simulink model "uncontrolled_case"  (R2020b)
settings: Solver=ode15s  StartTime=0.0  StopTime=T  MaxStep=0.01  RelTol=1e-3
values from neighbouring files (symbols this model uses):
  a1A = 0.5    [sim_D_FB_J.m]
  a1B = 0.5    [sim_D_FB_J.m]
  a2A = 0.5    [sim_D_FB_J.m]
  a2B = 0.5    [sim_D_FB_J.m]
  a3A = 0.5    [sim_D_FB_J.m]
  a3B = 0.5    [sim_D_FB_J.m]
  friction = [fv1p fv2p fv1A fv2A fv3A fv1B fv2B fv3B]    [sim_second_arm_compensation.m]    (also in sim_second_arm_compensation2.m; sim_second_arm_compensation3.m)
  fv1A = 0    [sim_D_FB_J.m]
  fv1B = 0    [sim_D_FB_J.m]
  fv2A = 0    [sim_D_FB_J.m]
  fv2B = 0    [sim_D_FB_J.m]
  fv3A = 0    [sim_D_FB_J.m]
  fv3B = 0    [sim_D_FB_J.m]
  g = [0 -g0 0]'    [sim_second_arm_compensation.m]    (also in sim_second_arm_compensation2.m; sim_second_arm_compensation3.m)
  info = struct('n_joints', n_joints,                'n_links', n_links,                'n_ee', n_ee,                'current_frame_index',    [1  2 3 4 5 6 7  8 9 10],                'previous_frame_index',   [0  1 2 3 4 2 6  7 5  8],                'next_frame_index',       [2 36 4 5 9 7 8 10 0  0],                'next_frame_type',        [0  1 0 0 0 0 0  0 0  0],                'previous_joint_index',  ...(+449 chars)    [sim_second_arm_compensation.m]    (also in sim_second_arm_compensation2.m; sim_second_arm_compensation3.m)
  Kd = 5*eye(6)    [sim_D_FB_J.m]    (also in sim_second_arm_compensation.m; sim_second_arm_compensation2.m; sim_second_arm_compensation3.m = diag([5 5 5 1 1 1]))
  Kp = 5*eye(6)    [sim_D_FB_J.m]    (also in sim_second_arm_compensation.m; sim_second_arm_compensation2.m; sim_second_arm_compensation3.m = diag([5 5 5 1 1 1]))
  L = 3    [sim_D_FB_J.m]
  m_base = 100    [sim_D_FB_J.m]
  m_cavo = 45    [sim_D_FB_J.m]
  ml1A = 5    [sim_D_FB_J.m]
  ml1B = 5    [sim_D_FB_J.m]
  ml2A = 5    [sim_D_FB_J.m]
  ml2B = 5    [sim_D_FB_J.m]
  ml3A = 5    [sim_D_FB_J.m]
  ml3B = 5    [sim_D_FB_J.m]
  offA = -0.25    [sim_D_FB_J.m]
  offB = 0.25    [sim_D_FB_J.m]
  th1A_0 = -pi/2    (= -1.57079632679)    [sim_D_FB_J.m]    (also in sim_second_arm_compensation.m = 0; sim_second_arm_compensation2.m = 0; sim_second_arm_compensation3.m = -0.523598775598)
  th1B_0 = -pi/2    (= -1.57079632679)    [sim_D_FB_J.m]    (also in sim_second_arm_compensation.m = 0; sim_second_arm_compensation2.m = 0; sim_second_arm_compensation3.m = 0.523598775598)
  th2A_0 = -pi/8    (= -0.392699081699)    [sim_D_FB_J.m]    (also in sim_second_arm_compensation.m; sim_second_arm_compensation2.m; sim_second_arm_compensation3.m = 0.523598775598)
  th2B_0 = pi/8    (= 0.392699081699)    [sim_D_FB_J.m]    (also in sim_second_arm_compensation.m; sim_second_arm_compensation2.m; sim_second_arm_compensation3.m = -0.523598775598)
  th3A_0 = -pi/8    (= -0.392699081699)    [sim_D_FB_J.m]    (also in sim_second_arm_compensation.m; sim_second_arm_compensation2.m; sim_second_arm_compensation3.m = 0.523598775598)
  th3B_0 = pi/8    (= 0.392699081699)    [sim_D_FB_J.m]    (also in sim_second_arm_compensation.m; sim_second_arm_compensation2.m; sim_second_arm_compensation3.m = -0.523598775598)
undefined symbols (not defined in the file or in its folder): D, m_cables, m_carroponte, m_crane, m_platform, X, Y, Z
libraries: sm_lib x173, nesl_utility x62
(part 1 of 4)
settings Model: Creator=giank  LastModifiedBy=giank
settings ExplorerConfigSet: InternalSimMechanicsExplorerSettings="<ExplorerConfiguration><canonicalview>default</canonicalview><AnimationSetting><BasePlaybackSpeed>1.0</BasePlaybackSpeed><PlaybackSpeedFactor>1.0</PlaybackSpeedFactor></AnimationSetting><TilePanel><TileInfo><Tiles Columns=\"1\" Count=\"1\" Rows=\"1\"><Column Weight=\"1\"/><Row Weight=\"1\"/><Tile Height=\"1\" Width=\"1\" X=\"0\" Y=\"0\"/></Tiles></TileInfo><SceneInfo><SceneViewer><BGColor><R>0.60000002384185791</R><G>0.60000002384185791</G><B>0.60000002384185791</B></BGColor><Camera><DoPerspective>off</DoPerspective><Position><X>0</X><Y>-2.20697786868344448</Y><Z>3.0855161704941283</Z></Position><Center><X>0</X><Y>-2.20697786868344448</Y><Z>9.61255199882771194e-08</Z></Center><Up><X>0</X><Y>1</Y><Z>-0</Z></Up><ViewLimDist>1</ViewLimDist><YLim>2.29378715991973881</YLim><XLim>3.51908945507964566</XLim></Camera></SceneViewer></SceneInfo></TilePanel><MechEditorPanel><Cameras/><GfxPanelCameraMap/><VideoCreator><PlaybackSpeedRatio>1.0</PlaybackSpeedRatio><FrameRate>30</FrameRate><VideoFormat>Motion JPEG AVI</VideoFormat><FrameSize>auto</FrameSize></VideoCreator></MechEditorPanel></ExplorerConfiguration>"

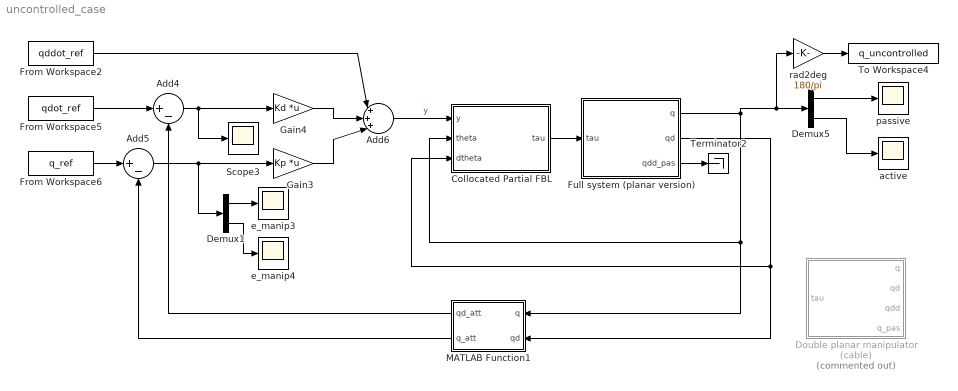
== system uncontrolled_case ==
  Add4 : Sum  Inputs=|+-
  Add5 : Sum  Inputs=|+-
  Add6 : Sum  Inputs=|+++|
  Collocated Partial FBL : MATLAB Function  TreatAsAtomicUnit=on
  Demux1 : Demux  Outputs=[3 3]
  Demux5 : Demux  Outputs=[2 6]
  Double planar manipulator (cable) : Subsystem  Commented=on
  From Workspace2 : FromWorkspace  VariableName=qddot_ref
  From Workspace5 : FromWorkspace  VariableName=qdot_ref
  From Workspace6 : FromWorkspace  VariableName=q_ref
  Full system (planar version) : Subsystem
  Gain3 : Gain  Gain=Kp  Multiplication=Matrix(K*u)
  Gain4 : Gain  Gain=Kd  Multiplication=Matrix(K*u)
  MATLAB Function1 : MATLAB Function  TreatAsAtomicUnit=on
  Scope3 : Scope
  Terminator2 : Terminator
  To Workspace4 : ToWorkspace  VariableName=q_uncontrolled  SaveFormat=Timeseries  SampleTime=-1
  active : Scope
  e_manip3 : Scope
  e_manip4 : Scope
  passive : Scope
  rad2deg : Gain  Gain=180/pi
  wires:
  From Workspace5/1 -> Add4/1
  MATLAB Function1/1(qd_att) -> Add4/2
  From Workspace6/1 -> Add5/1
  Add4/1 -> Scope3/1, Gain4/1
  Gain3/1 -> Add6/3
  Gain4/1 -> Add6/2
  Collocated Partial FBL/1(tau) -> Full system (planar version)/1(tau)
  MATLAB Function1/2(q_att) -> Add5/2
  Full system (planar version)/2(qd) -> Collocated Partial FBL/3(dtheta), MATLAB Function1/2(qd)
  Demux5/2 -> active/1
  Full system (planar version)/3(qdd_pas) -> Terminator2/1
  From Workspace2/1 -> Add6/1
  Demux5/1 -> passive/1
  Add6/1 -> Collocated Partial FBL/1(y)  "y"
  Full system (planar version)/1(q) -> rad2deg/1, Demux5/1, MATLAB Function1/1(q), Collocated Partial FBL/2(theta)
  Demux1/1 -> e_manip3/1
  Demux1/2 -> e_manip4/1
  Add5/1 -> Demux1/1, Gain3/1
  rad2deg/1 -> To Workspace4/1

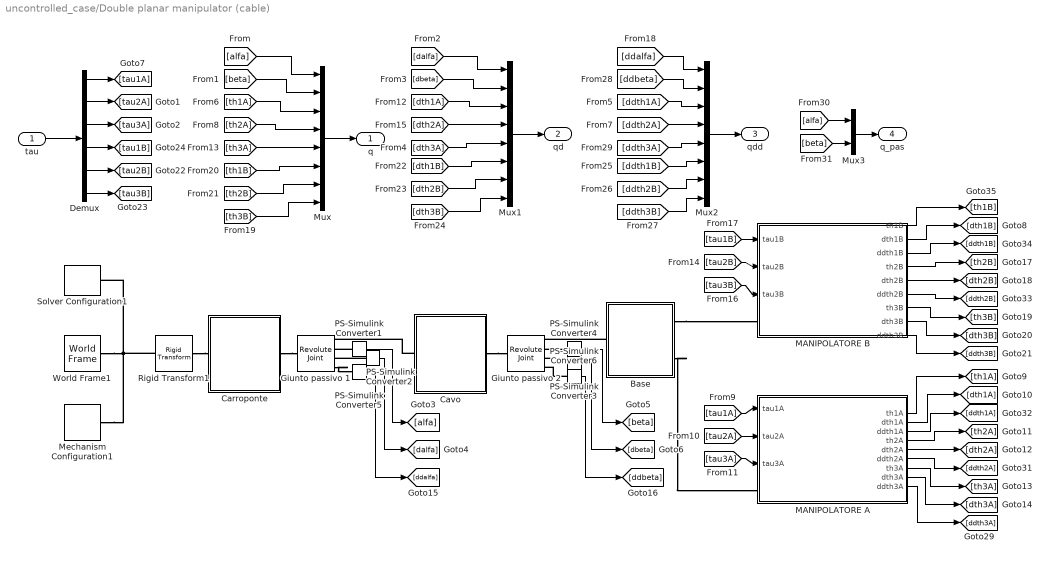
== system uncontrolled_case/Double planar manipulator (cable) ==
  tau : Inport
  Base : Subsystem  mask{L=1.2, W=0.15, H=0.15, m=m_base, rgb=[0.80 0.45 0]}
      mask prompts: L "Lenght (m)"; W "Width (m)"; H "Thickness (m)"; m "Mass (kg)"; rgb "Color [R G B]"
  Carroponte : Subsystem
  Cavo : Subsystem  mask{L=L, W=0.05, H=0.05, m=m_cavo, rgb=[0.3 0.3 0.3]}
      mask prompts: L "Lenght (m)"; W "Width (m)"; H "Thickness (m)"; m "Mass (kg)"; rgb "Color [R G B]"
  Demux : Demux  Outputs=6
  Giunto passivo 1 : sm_lib/Joints/Revolute Joint  JointMode=Normal  SenseConstraintForce=off  SenseConstraintForceX=off  SenseConstraintForceY=off  SenseConstraintForceZ=off  SenseConstraintTorque=off  SenseConstraintTorqueX=off  SenseConstraintTorqueY=off  SenseConstraintTorqueZ=off  SenseTotalForce=off  SenseTotalForceX=off  SenseTotalForceY=off  SenseTotalForceZ=off  SenseTotalTorque=off  SenseTotalTorqueX=off  SenseTotalTorqueY=off  SenseTotalTorqueZ=off  CompositeWrenchDir=FollowerOnBase  CompositeWrenchFrame=BaseFrame  EquilibriumPosition=0  EquilibriumPositionUnits=deg  SpringStiffness=0  SpringStiffnessUnits=N*m/deg  DampingCoefficient=fv1p  DampingCoefficientUnits=N*m/(rad/s)  TorqueActuationMode=NoTorque  MotionActuationMode=ComputedMotion  SensePosition=on  SenseVelocity=on  SenseAcceleration=on  SenseTorqueForce=off  SenseLowerLimitTorqueForce=off  SenseUpperLimitTorqueForce=off  LowerLimitSpecify=off  LowerLimitBound=-90  LowerLimitBoundUnits=deg  LowerLimitStiffness=1e4  LowerLimitStiffnessUnits=N*m/deg  LowerLimitDamping=10  LowerLimitDampingUnits=N*m/(deg/s)  LowerLimitTransitionRegionWidth=0.1  LowerLimitTransitionRegionWidthUnits=deg  UpperLimitSpecify=off  UpperLimitBound=90  UpperLimitBoundUnits=deg  UpperLimitStiffness=1e4  UpperLimitStiffnessUnits=N*m/deg  UpperLimitDamping=10  UpperLimitDampingUnits=N*m/(deg/s)  UpperLimitTransitionRegionWidth=0.1  UpperLimitTransitionRegionWidthUnits=deg  PositionTargetSpecify=on  PositionTargetPriority=High  PositionTargetValue=alfa_0  PositionTargetValueUnits=rad  VelocityTargetSpecify=off  VelocityTargetPriority=High  VelocityTargetValue=0  VelocityTargetValueUnits=deg/s
  Giunto passivo 2 : sm_lib/Joints/Revolute Joint  JointMode=Normal  SenseConstraintForce=off  SenseConstraintForceX=off  SenseConstraintForceY=off  SenseConstraintForceZ=off  SenseConstraintTorque=off  SenseConstraintTorqueX=off  SenseConstraintTorqueY=off  SenseConstraintTorqueZ=off  SenseTotalForce=off  SenseTotalForceX=off  SenseTotalForceY=off  SenseTotalForceZ=off  SenseTotalTorque=off  SenseTotalTorqueX=off  SenseTotalTorqueY=off  SenseTotalTorqueZ=off  CompositeWrenchDir=FollowerOnBase  CompositeWrenchFrame=BaseFrame  EquilibriumPosition=0  EquilibriumPositionUnits=deg  SpringStiffness=0  SpringStiffnessUnits=N*m/deg  DampingCoefficient=fv2p  DampingCoefficientUnits=N*m/(rad/s)  TorqueActuationMode=NoTorque  MotionActuationMode=ComputedMotion  SensePosition=on  SenseVelocity=on  SenseAcceleration=on  SenseTorqueForce=off  SenseLowerLimitTorqueForce=off  SenseUpperLimitTorqueForce=off  LowerLimitSpecify=off  LowerLimitBound=-90  LowerLimitBoundUnits=deg  LowerLimitStiffness=1e4  LowerLimitStiffnessUnits=N*m/deg  LowerLimitDamping=10  LowerLimitDampingUnits=N*m/(deg/s)  LowerLimitTransitionRegionWidth=0.1  LowerLimitTransitionRegionWidthUnits=deg  UpperLimitSpecify=off  UpperLimitBound=90  UpperLimitBoundUnits=deg  UpperLimitStiffness=1e4  UpperLimitStiffnessUnits=N*m/deg  UpperLimitDamping=10  UpperLimitDampingUnits=N*m/(deg/s)  UpperLimitTransitionRegionWidth=0.1  UpperLimitTransitionRegionWidthUnits=deg  PositionTargetSpecify=on  PositionTargetPriority=High  PositionTargetValue=beta_0  PositionTargetValueUnits=rad  VelocityTargetSpecify=off  VelocityTargetPriority=High  VelocityTargetValue=0  VelocityTargetValueUnits=deg/s
  MANIPOLATORE A : Subsystem  mask{th1_0=th1A_0, th2_0=th2A_0, th3_0=th3A_0, fv1=fv1A, fv2=fv2A, fv3=fv3A, a1=a1A, a2=a2A, a3=a3A, ml1=ml1A, ml2=ml2A, ml3=ml3A}
      mask prompts: th1_0 "th1_0 (rad)"; th2_0 "th2_0 (rad)"; th3_0 "th3_0 (rad)"; fv1 "Damping coeff. joint 1 (N*m/(rad/s))"; fv2 "Damping coeff. joint 2 (N*m/(rad/s))"; fv3 "Damping coeff. joint 3 (N*m/(rad/s))"; a1 "a1 (m)"; a2 "a2 (m)"; a3 "a3 (m)"; ml1 "ml1 (kg)"; ml2 "ml2 (kg)"; ml3 "ml3 (kg)"
  MANIPOLATORE B : Subsystem  mask{th1_0=th1B_0, th2_0=th2B_0, th3_0=th3B_0, fv1=fv1B, fv2=fv2B, fv3=fv3B, a1=a1B, a2=a2B, a3=a3B, ml1=ml1B, ml2=ml2B, ml3=ml3B}
      mask prompts: th1_0 "th1_0 (rad)"; th2_0 "th2_0 (rad)"; th3_0 "th3_0 (rad)"; fv1 "Damping coeff. joint 1 (N*m/(rad/s))"; fv2 "Damping coeff. joint 2 (N*m/(rad/s))"; fv3 "Damping coeff. joint 3 (N*m/(rad/s))"; a1 "a1 (m)"; a2 "a2 (m)"; a3 "a3 (m)"; ml1 "ml1 (kg)"; ml2 "ml2 (kg)"; ml3 "ml3 (kg)"
  Mechanism Configuration1 : sm_lib/Utilities/Mechanism Configuration  UniformGravity=Constant  GravityVector=[0 -9.81 0]  GravityVectorUnits=m/s^2  GravityUnits=m/s^2  LinearizationDelta=0.001  JointModeTransitionNonlinearIterations=2
  Mux : Mux  Inputs=8
  Mux1 : Mux  Inputs=8
  Mux2 : Mux  Inputs=8
  Mux3 : Mux  Inputs=2
  PS-Simulink Converter{1..6} (6 alike) : nesl_utility/PS-Simulink Converter  PhysicalDomain=network_engine_domain  SubClassName=ps_output  LeftPortType=input  RightPortType=output  PseudoPeriodic=off  Frequencies=[]  Unit=inherit  AffineConversion=off
  Rigid Transform1 : sm_lib/Frames and Transforms/Rigid Transform  TranslationMethod=StandardAxis  TranslationStandardOffset=9.5  TranslationLengthUnit=cm  TranslationStandardAxis=-Y  TranslationCartesianOffset=[0 0 0]  TranslationROffset=0  TranslationROffsetUnits=m  TranslationZOffset=0  TranslationZOffsetUnits=m  TranslationThetaOffset=0  TranslationThetaOffsetUnits=deg  RotationMethod=StandardAxis  RotationAngleUnits=deg  RotationStandardAxis=+Y  RotationAngle=90  RotationArbitraryAxis=[0 0 1]  FollAlignAxisA=+X  BaseAlignAxisA=+Y  FollAlignAxisB=+Y  BaseAlignAxisB=+Z  RotationSequenceAxes=FollowerAxes  RotationSequence=XYX  RotationSequenceAngles=[0 0 0]  RotationSequenceAnglesUnits=deg  RotationMatrix=[1 0 0; 0 1 0; 0 0 1]
  Solver Configuration1 : nesl_utility/Solver Configuration  PhysicalDomain=network_engine_domain  SubClassName=solver  LeftPortType=input  RightPortType=generic  Tones=[]  Harmonics=[]  SimulateNoise=off  Profile=off  UseLocalSampling=off  EnableSwitchedLinearOptims=on  FrequencyDomain=off  UseCCode=off  RelTol=0.001  AbsTol=1e-06  MinStep=1e-09  ToWorkspace=off  RevertToSquareIcSolve=off  NumHomotopyIterations=100  PhasorMode=off  PhasorModeNumHarmonics=1  DoDC=off  ResidualTolerance=1e-09  UseLocalSolver=off  LocalSolverChoice=NE_BACKWARD_EULER_ADVANCER  LocalSolverSampleTime=0.001  DoFixedCost=off  MaxNonlinIter=3  MaxModeIter=2  ComputeImpulses=off  ImpulseIterations=2  LinearAlgebra=Sparse  EquationFormulation=NE_TIME_EF  DelaysMemoryBudget=1024  AutomaticFiltering=on  FilteringTimeConstant=0.001  PartitionStorageMethod=AS_NEEDED  PartitionMemoryBudget=1024  PartitionMethod=FAST
  World Frame1 : sm_lib/Frames and Transforms/World Frame
  q : Outport
  qd : Outport  Port=2
  qdd : Outport  Port=3
  q_pas : Outport  Port=4
  wires:
  Mux/1 -> q/1
  PS-Simulink Converter1/1 -> [alfa]
  PS-Simulink Converter2/1 -> [dalfa]
  PS-Simulink Converter4/1 -> [beta]
  PS-Simulink Converter3/1 -> [dbeta]
  tau/1 -> Demux/1
  Mux1/1 -> qd/1
  Demux/1 -> [tau1A]
  Demux/3 -> [tau3A]
  Demux/2 -> [tau2A]
  Demux/4 -> [tau1B]
  Demux/5 -> [tau2B]
  [beta] -> Mux/2
  [alfa] -> Mux/1
  [th1A] -> Mux/3
  [th2A] -> Mux/4
  [th3A] -> Mux/5
  [th1B] -> Mux/6
  [th2B] -> Mux/7
  [th3B] -> Mux/8
  [dalfa] -> Mux1/1
  [dbeta] -> Mux1/2
  [dth1A] -> Mux1/3
  [dth2A] -> Mux1/4
  [dth3A] -> Mux1/5
  [dth1B] -> Mux1/6
  [dth2B] -> Mux1/7
  [dth3B] -> Mux1/8
  Demux/6 -> [tau3B]
  PS-Simulink Converter5/1 -> [ddalfa]
  PS-Simulink Converter6/1 -> [ddbeta]
  [ddalfa] -> Mux2/1
  Mux2/1 -> qdd/1
  [ddth1A] -> Mux2/3
  [ddth3B] -> Mux2/8
  [ddth2B] -> Mux2/7
  [ddth2A] -> Mux2/4
  [ddbeta] -> Mux2/2
  [ddth1B] -> Mux2/6
  [ddth3A] -> Mux2/5
  [alfa] -> Mux3/1
  [beta] -> Mux3/2
  Mux3/1 -> q_pas/1
  MANIPOLATORE A/1(th1A) -> [th1A]
  [tau3B] -> MANIPOLATORE B/3(tau3B)
  MANIPOLATORE B/1(th1B) -> [th1B]
  [tau1B] -> MANIPOLATORE B/1(tau1B)
  [tau2B] -> MANIPOLATORE B/2(tau2B)
  MANIPOLATORE B/4(th2B) -> [th2B]
  MANIPOLATORE B/5(dth2B) -> [dth2B]
  MANIPOLATORE B/7(th3B) -> [th3B]
  MANIPOLATORE A/5(dth2A) -> [dth2A]
  [tau2A] -> MANIPOLATORE A/2(tau2A)
  MANIPOLATORE A/4(th2A) -> [th2A]
  MANIPOLATORE A/8(dth3A) -> [dth3A]
  MANIPOLATORE A/9(ddth3A) -> [ddth3A]
  MANIPOLATORE B/6(ddth2B) -> [ddth2B]
  [tau1A] -> MANIPOLATORE A/1(tau1A)
  MANIPOLATORE A/7(th3A) -> [th3A]
  MANIPOLATORE B/8(dth3B) -> [dth3B]
  MANIPOLATORE B/9(ddth3B) -> [ddth3B]
  MANIPOLATORE A/2(dth1A) -> [dth1A]
  MANIPOLATORE A/6(ddth2A) -> [ddth2A]
  [tau3A] -> MANIPOLATORE A/3(tau3A)
  MANIPOLATORE B/2(dth1B) -> [dth1B]
  MANIPOLATORE B/3(ddth1B) -> [ddth1B]
  MANIPOLATORE A/3(ddth1A) -> [ddth1A]
  connections:
  Rigid Transform1/LConn1 -- Mechanism Configuration1/RConn1 -- World Frame1/RConn1 -- Solver Configuration1/RConn1
  Cavo/LConn1 -- Giunto passivo 1/RConn1
  Rigid Transform1/RConn1 -- Carroponte/LConn1
  Carroponte/RConn1 -- Giunto passivo 1/LConn1
  Cavo/RConn1 -- Giunto passivo 2/LConn1
  Base/LConn1 -- Giunto passivo 2/RConn1
  PS-Simulink Converter1/LConn1 -- Giunto passivo 1/RConn2
  PS-Simulink Converter4/LConn1 -- Giunto passivo 2/RConn2
  PS-Simulink Converter3/LConn1 -- Giunto passivo 2/RConn3
  PS-Simulink Converter2/LConn1 -- Giunto passivo 1/RConn3
  Giunto passivo 1/RConn4 -- PS-Simulink Converter5/LConn1
  PS-Simulink Converter6/LConn1 -- Giunto passivo 2/RConn4
  Base/RConn1 -- MANIPOLATORE B/LConn1
  Base/RConn2 -- MANIPOLATORE A/LConn1

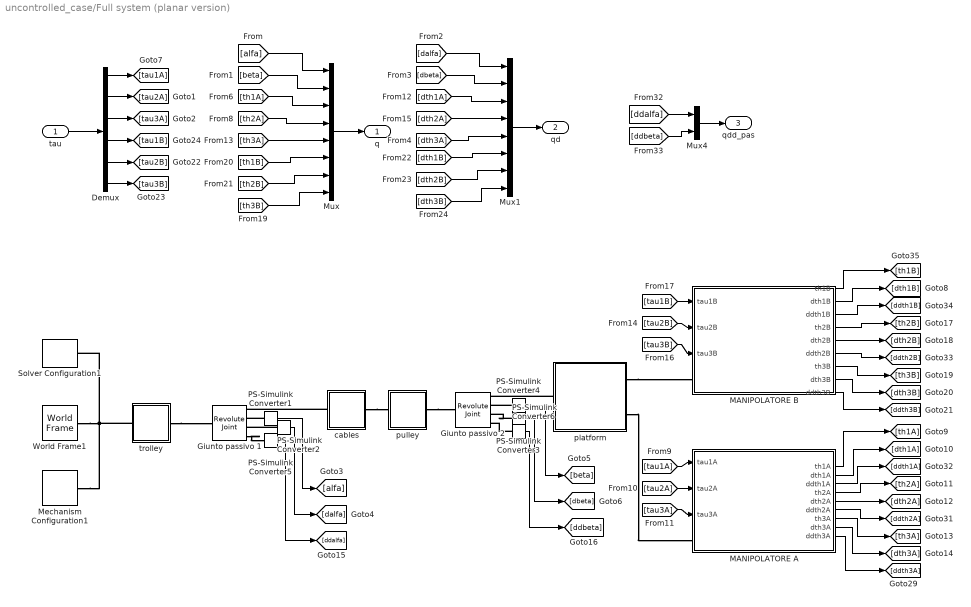
== system uncontrolled_case/Full system (planar version) ==
  tau : Inport
  Demux : Demux  Outputs=6
  Giunto passivo 1 : sm_lib/Joints/Revolute Joint  JointMode=Normal  SenseConstraintForce=off  SenseConstraintForceX=off  SenseConstraintForceY=off  SenseConstraintForceZ=off  SenseConstraintTorque=off  SenseConstraintTorqueX=off  SenseConstraintTorqueY=off  SenseConstraintTorqueZ=off  SenseTotalForce=off  SenseTotalForceX=off  SenseTotalForceY=off  SenseTotalForceZ=off  SenseTotalTorque=off  SenseTotalTorqueX=off  SenseTotalTorqueY=off  SenseTotalTorqueZ=off  CompositeWrenchDir=FollowerOnBase  CompositeWrenchFrame=BaseFrame  EquilibriumPosition=0  EquilibriumPositionUnits=deg  SpringStiffness=0  SpringStiffnessUnits=N*m/deg  DampingCoefficient=fv1p  DampingCoefficientUnits=N*m/(rad/s)  TorqueActuationMode=NoTorque  MotionActuationMode=ComputedMotion  SensePosition=on  SenseVelocity=on  SenseAcceleration=on  SenseTorqueForce=off  SenseLowerLimitTorqueForce=off  SenseUpperLimitTorqueForce=off  LowerLimitSpecify=off  LowerLimitBound=-90  LowerLimitBoundUnits=deg  LowerLimitStiffness=1e4  LowerLimitStiffnessUnits=N*m/deg  LowerLimitDamping=10  LowerLimitDampingUnits=N*m/(deg/s)  LowerLimitTransitionRegionWidth=0.1  LowerLimitTransitionRegionWidthUnits=deg  UpperLimitSpecify=off  UpperLimitBound=90  UpperLimitBoundUnits=deg  UpperLimitStiffness=1e4  UpperLimitStiffnessUnits=N*m/deg  UpperLimitDamping=10  UpperLimitDampingUnits=N*m/(deg/s)  UpperLimitTransitionRegionWidth=0.1  UpperLimitTransitionRegionWidthUnits=deg  PositionTargetSpecify=on  PositionTargetPriority=High  PositionTargetValue=alfa_0  PositionTargetValueUnits=rad  VelocityTargetSpecify=off  VelocityTargetPriority=High  VelocityTargetValue=0  VelocityTargetValueUnits=deg/s
  Giunto passivo 2 : sm_lib/Joints/Revolute Joint  JointMode=Normal  SenseConstraintForce=off  SenseConstraintForceX=off  SenseConstraintForceY=off  SenseConstraintForceZ=off  SenseConstraintTorque=off  SenseConstraintTorqueX=off  SenseConstraintTorqueY=off  SenseConstraintTorqueZ=off  SenseTotalForce=off  SenseTotalForceX=off  SenseTotalForceY=off  SenseTotalForceZ=off  SenseTotalTorque=off  SenseTotalTorqueX=off  SenseTotalTorqueY=off  SenseTotalTorqueZ=off  CompositeWrenchDir=FollowerOnBase  CompositeWrenchFrame=BaseFrame  EquilibriumPosition=0  EquilibriumPositionUnits=deg  SpringStiffness=0  SpringStiffnessUnits=N*m/deg  DampingCoefficient=fv2p  DampingCoefficientUnits=N*m/(rad/s)  TorqueActuationMode=NoTorque  MotionActuationMode=ComputedMotion  SensePosition=on  SenseVelocity=on  SenseAcceleration=on  SenseTorqueForce=off  SenseLowerLimitTorqueForce=off  SenseUpperLimitTorqueForce=off  LowerLimitSpecify=off  LowerLimitBound=-90  LowerLimitBoundUnits=deg  LowerLimitStiffness=1e4  LowerLimitStiffnessUnits=N*m/deg  LowerLimitDamping=10  LowerLimitDampingUnits=N*m/(deg/s)  LowerLimitTransitionRegionWidth=0.1  LowerLimitTransitionRegionWidthUnits=deg  UpperLimitSpecify=off  UpperLimitBound=90  UpperLimitBoundUnits=deg  UpperLimitStiffness=1e4  UpperLimitStiffnessUnits=N*m/deg  UpperLimitDamping=10  UpperLimitDampingUnits=N*m/(deg/s)  UpperLimitTransitionRegionWidth=0.1  UpperLimitTransitionRegionWidthUnits=deg  PositionTargetSpecify=on  PositionTargetPriority=High  PositionTargetValue=beta_0  PositionTargetValueUnits=rad  VelocityTargetSpecify=off  VelocityTargetPriority=High  VelocityTargetValue=0  VelocityTargetValueUnits=deg/s
  MANIPOLATORE A : Subsystem  mask{th1_0=th1A_0, th2_0=th2A_0, th3_0=th3A_0, fv1=fv1A, fv2=fv2A, fv3=fv3A, a1=a1A, a2=a2A, a3=a3A, ml1=ml1A, ml2=ml2A, ml3=ml3A}
      mask prompts: th1_0 "th1_0 (rad)"; th2_0 "th2_0 (rad)"; th3_0 "th3_0 (rad)"; fv1 "Damping coeff. joint 1 (N*m/(rad/s))"; fv2 "Damping coeff. joint 2 (N*m/(rad/s))"; fv3 "Damping coeff. joint 3 (N*m/(rad/s))"; a1 "a1 (m)"; a2 "a2 (m)"; a3 "a3 (m)"; ml1 "ml1 (kg)"; ml2 "ml2 (kg)"; ml3 "ml3 (kg)"
  MANIPOLATORE B : Subsystem  mask{th1_0=th1B_0, th2_0=th2B_0, th3_0=th3B_0, fv1=fv1B, fv2=fv2B, fv3=fv3B, a1=a1B, a2=a2B, a3=a3B, ml1=ml1B, ml2=ml2B, ml3=ml3B}
      mask prompts: th1_0 "th1_0 (rad)"; th2_0 "th2_0 (rad)"; th3_0 "th3_0 (rad)"; fv1 "Damping coeff. joint 1 (N*m/(rad/s))"; fv2 "Damping coeff. joint 2 (N*m/(rad/s))"; fv3 "Damping coeff. joint 3 (N*m/(rad/s))"; a1 "a1 (m)"; a2 "a2 (m)"; a3 "a3 (m)"; ml1 "ml1 (kg)"; ml2 "ml2 (kg)"; ml3 "ml3 (kg)"
  Mechanism Configuration1 : sm_lib/Utilities/Mechanism Configuration  UniformGravity=Constant  GravityVector=[0 -9.81 0]  GravityVectorUnits=m/s^2  GravityUnits=m/s^2  LinearizationDelta=0.001  JointModeTransitionNonlinearIterations=2
  Mux : Mux  Inputs=8
  Mux1 : Mux  Inputs=8
  Mux4 : Mux  Inputs=2
  PS-Simulink Converter{1..6} (6 alike) : nesl_utility/PS-Simulink Converter  PhysicalDomain=network_engine_domain  SubClassName=ps_output  LeftPortType=input  RightPortType=output  PseudoPeriodic=off  Frequencies=[]  Unit=inherit  AffineConversion=off
  Solver Configuration1 : nesl_utility/Solver Configuration  PhysicalDomain=network_engine_domain  SubClassName=solver  LeftPortType=input  RightPortType=generic  Tones=[]  Harmonics=[]  SimulateNoise=off  Profile=off  UseLocalSampling=off  EnableSwitchedLinearOptims=on  FrequencyDomain=off  UseCCode=off  RelTol=0.001  AbsTol=1e-06  MinStep=1e-09  ToWorkspace=off  RevertToSquareIcSolve=off  NumHomotopyIterations=100  PhasorMode=off  PhasorModeNumHarmonics=1  DoDC=off  ResidualTolerance=1e-09  UseLocalSolver=off  LocalSolverChoice=NE_BACKWARD_EULER_ADVANCER  LocalSolverSampleTime=0.001  DoFixedCost=off  MaxNonlinIter=3  MaxModeIter=2  ComputeImpulses=off  ImpulseIterations=2  LinearAlgebra=Sparse  EquationFormulation=NE_TIME_EF  DelaysMemoryBudget=1024  AutomaticFiltering=on  FilteringTimeConstant=0.001  PartitionStorageMethod=AS_NEEDED  PartitionMemoryBudget=1024  PartitionMethod=FAST
  World Frame1 : sm_lib/Frames and Transforms/World Frame
  cables : Subsystem
  platform : Subsystem
  pulley : Subsystem
  trolley : Subsystem
  q : Outport
  qd : Outport  Port=2
  qdd_pas : Outport  Port=3
  wires:
  Mux/1 -> q/1
  PS-Simulink Converter1/1 -> [alfa]
  PS-Simulink Converter2/1 -> [dalfa]
  PS-Simulink Converter4/1 -> [beta]
  PS-Simulink Converter3/1 -> [dbeta]
  tau/1 -> Demux/1
  Mux1/1 -> qd/1
  Demux/1 -> [tau1A]
  Demux/3 -> [tau3A]
  Demux/2 -> [tau2A]
  Demux/4 -> [tau1B]
  Demux/5 -> [tau2B]
  [beta] -> Mux/2
  [alfa] -> Mux/1
  [th1A] -> Mux/3
  [th2A] -> Mux/4
  [th3A] -> Mux/5
  [th1B] -> Mux/6
  [th2B] -> Mux/7
  [th3B] -> Mux/8
  [dalfa] -> Mux1/1
  [dbeta] -> Mux1/2
  [dth1A] -> Mux1/3
  [dth2A] -> Mux1/4
  [dth3A] -> Mux1/5
  [dth1B] -> Mux1/6
  [dth2B] -> Mux1/7
  [dth3B] -> Mux1/8
  Demux/6 -> [tau3B]
  PS-Simulink Converter5/1 -> [ddalfa]
  PS-Simulink Converter6/1 -> [ddbeta]
  MANIPOLATORE A/1(th1A) -> [th1A]
  [tau3B] -> MANIPOLATORE B/3(tau3B)
  MANIPOLATORE B/1(th1B) -> [th1B]
  [tau1B] -> MANIPOLATORE B/1(tau1B)
  [tau2B] -> MANIPOLATORE B/2(tau2B)
  MANIPOLATORE B/4(th2B) -> [th2B]
  MANIPOLATORE B/5(dth2B) -> [dth2B]
  MANIPOLATORE B/7(th3B) -> [th3B]
  MANIPOLATORE A/5(dth2A) -> [dth2A]
  [tau2A] -> MANIPOLATORE A/2(tau2A)
  MANIPOLATORE A/4(th2A) -> [th2A]
  MANIPOLATORE A/8(dth3A) -> [dth3A]
  MANIPOLATORE A/9(ddth3A) -> [ddth3A]
  MANIPOLATORE B/6(ddth2B) -> [ddth2B]
  [tau1A] -> MANIPOLATORE A/1(tau1A)
  MANIPOLATORE A/7(th3A) -> [th3A]
  MANIPOLATORE B/8(dth3B) -> [dth3B]
  MANIPOLATORE B/9(ddth3B) -> [ddth3B]
  MANIPOLATORE A/2(dth1A) -> [dth1A]
  MANIPOLATORE A/6(ddth2A) -> [ddth2A]
  [tau3A] -> MANIPOLATORE A/3(tau3A)
  MANIPOLATORE B/2(dth1B) -> [dth1B]
  MANIPOLATORE B/3(ddth1B) -> [ddth1B]
  MANIPOLATORE A/3(ddth1A) -> [ddth1A]
  Mux4/1 -> qdd_pas/1
  [ddbeta] -> Mux4/2
  [ddalfa] -> Mux4/1
  connections:
  Mechanism Configuration1/RConn1 -- trolley/LConn1 -- World Frame1/RConn1 -- Solver Configuration1/RConn1
  cables/LConn1 -- Giunto passivo 1/RConn1
  trolley/RConn1 -- Giunto passivo 1/LConn1
  platform/LConn1 -- Giunto passivo 2/RConn1
  PS-Simulink Converter1/LConn1 -- Giunto passivo 1/RConn2
  PS-Simulink Converter4/LConn1 -- Giunto passivo 2/RConn2
  PS-Simulink Converter3/LConn1 -- Giunto passivo 2/RConn3
  PS-Simulink Converter2/LConn1 -- Giunto passivo 1/RConn3
  Giunto passivo 1/RConn4 -- PS-Simulink Converter5/LConn1
  PS-Simulink Converter6/LConn1 -- Giunto passivo 2/RConn4
  platform/RConn1 -- MANIPOLATORE B/LConn1
  platform/RConn2 -- MANIPOLATORE A/LConn1
  cables/RConn1 -- pulley/LConn1
  pulley/RConn1 -- Giunto passivo 2/LConn1

== system uncontrolled_case/Double planar manipulator (cable)/Base ==
  Brick Solid : sm_lib/Body Elements/Brick Solid  GraphicAmbientColor=[0.15 0.15 0.15 1.0]  BasedOnType=Mass  BrickDimensions=[L W H]  BrickDimensionUnits=m  CenterOfMass=[0 0 0]  CenterOfMassUnits=m  GraphicDiffuseColor=rgb  Density=1000  DensityUnits=kg/m^3  DoExposeReferenceFrame=on  GraphicEmissiveColor=[0.0 0.0 0.0 1.0]  ExportEntireGeometry=off  SerializedFrames=<Frames/>  MarkerShape=Sphere  MarkerSize=10  GraphicType=FromGeometry  InertiaType=CalculateFromGeometry  Mass=m  MassUnits=kg  MomentsOfInertia=[1 1 1]  MomentsOfInertiaUnits=kg*m^2  GraphicOpacity=1.0  ProductsOfInertia=[0 0 0]  ProductsOfInertiaUnits=kg*m^2  GraphicShininess=75  GraphicSpecularColor=[0.5 0.5 0.5 1.0]  GraphicVisPropType=SimpleVisualProperties
  Rigid Transform1 : sm_lib/Frames and Transforms/Rigid Transform  TranslationMethod=Cartesian  TranslationStandardOffset=4  TranslationLengthUnit=m  TranslationStandardAxis=-Y  TranslationCartesianOffset=[offB 0 0]  TranslationROffset=0  TranslationROffsetUnits=m  TranslationZOffset=0  TranslationZOffsetUnits=m  TranslationThetaOffset=0  TranslationThetaOffsetUnits=deg  RotationMethod=StandardAxis  RotationAngleUnits=deg  RotationStandardAxis=+Z  RotationAngle=-90  RotationArbitraryAxis=[0 0 1]  FollAlignAxisA=+X  BaseAlignAxisA=+Y  FollAlignAxisB=+Y  BaseAlignAxisB=+Z  RotationSequenceAxes=FollowerAxes  RotationSequence=XYX  RotationSequenceAngles=[0 0 0]  RotationSequenceAnglesUnits=deg  RotationMatrix=[1 0 0; 0 1 0; 0 0 1]
  Rigid Transform2 : sm_lib/Frames and Transforms/Rigid Transform  TranslationMethod=Cartesian  TranslationStandardOffset=4  TranslationLengthUnit=m  TranslationStandardAxis=-Y  TranslationCartesianOffset=[offA 0 0]  TranslationROffset=0  TranslationROffsetUnits=m  TranslationZOffset=0  TranslationZOffsetUnits=m  TranslationThetaOffset=0  TranslationThetaOffsetUnits=deg  RotationMethod=StandardAxis  RotationAngleUnits=deg  RotationStandardAxis=+Z  RotationAngle=-90  RotationArbitraryAxis=[0 0 1]  FollAlignAxisA=+X  BaseAlignAxisA=+Y  FollAlignAxisB=+Y  BaseAlignAxisB=+Z  RotationSequenceAxes=FollowerAxes  RotationSequence=XYX  RotationSequenceAngles=[0 0 0]  RotationSequenceAnglesUnits=deg  RotationMatrix=[1 0 0; 0 1 0; 0 0 1]
  Conn1 : PMIOPort  Side=Left
  Conn3 : PMIOPort  Port=2  Side=Right
  Conn2 : PMIOPort  Port=3  Side=Right
  connections:
  Brick Solid/RConn1 -- Rigid Transform2/LConn1 -- Rigid Transform1/LConn1 -- Conn1/RConn1
  Rigid Transform2/RConn1 -- Conn2/RConn1
  Rigid Transform1/RConn1 -- Conn3/RConn1

== system uncontrolled_case/Double planar manipulator (cable)/Carroponte ==
  Base : sm_lib/Body Elements/Brick Solid  GraphicAmbientColor=[0.15 0.15 0.15 1.0]  BasedOnType=Mass  BrickDimensions=[80 15 15]  BrickDimensionUnits=cm  CenterOfMass=[0 0 0]  CenterOfMassUnits=m  GraphicDiffuseColor=[0.80 0.45 0]  Density=1000  DensityUnits=kg/m^3  DoExposeReferenceFrame=on  GraphicEmissiveColor=[0.0 0.0 0.0 1.0]  ExportEntireGeometry=off  SerializedFrames=<Frames/>  MarkerShape=Sphere  MarkerSize=10  GraphicType=FromGeometry  InertiaType=CalculateFromGeometry  Mass=m_carroponte  MassUnits=kg  MomentsOfInertia=[1 1 1]  MomentsOfInertiaUnits=kg*m^2  GraphicOpacity=1.0  ProductsOfInertia=[0 0 0]  ProductsOfInertiaUnits=kg*m^2  GraphicShininess=75  GraphicSpecularColor=[0.5 0.5 0.5 1.0]  GraphicVisPropType=SimpleVisualProperties
  Rigid Transform1 : sm_lib/Frames and Transforms/Rigid Transform  TranslationMethod=None  TranslationStandardOffset=4  TranslationLengthUnit=cm  TranslationStandardAxis=-Y  TranslationCartesianOffset=[0 0 0]  TranslationROffset=0  TranslationROffsetUnits=m  TranslationZOffset=0  TranslationZOffsetUnits=m  TranslationThetaOffset=0  TranslationThetaOffsetUnits=deg  RotationMethod=StandardAxis  RotationAngleUnits=deg  RotationStandardAxis=+Z  RotationAngle=-90  RotationArbitraryAxis=[0 0 1]  FollAlignAxisA=+X  BaseAlignAxisA=+Y  FollAlignAxisB=+Y  BaseAlignAxisB=+Z  RotationSequenceAxes=FollowerAxes  RotationSequence=XYX  RotationSequenceAngles=[0 0 0]  RotationSequenceAnglesUnits=deg  RotationMatrix=[1 0 0; 0 1 0; 0 0 1]
  Rigid Transform2 : sm_lib/Frames and Transforms/Rigid Transform  TranslationMethod=None  TranslationStandardOffset=4  TranslationLengthUnit=cm  TranslationStandardAxis=-Y  TranslationCartesianOffset=[0 0 0]  TranslationROffset=0  TranslationROffsetUnits=m  TranslationZOffset=0  TranslationZOffsetUnits=m  TranslationThetaOffset=0  TranslationThetaOffsetUnits=deg  RotationMethod=StandardAxis  RotationAngleUnits=deg  RotationStandardAxis=+Y  RotationAngle=-90  RotationArbitraryAxis=[0 0 1]  FollAlignAxisA=+X  BaseAlignAxisA=+Y  FollAlignAxisB=+Y  BaseAlignAxisB=+Z  RotationSequenceAxes=FollowerAxes  RotationSequence=XYX  RotationSequenceAngles=[0 0 0]  RotationSequenceAnglesUnits=deg  RotationMatrix=[1 0 0; 0 1 0; 0 0 1]
  Conn1 : PMIOPort  Side=Left
  Conn2 : PMIOPort  Port=2  Side=Right
  connections:
  Rigid Transform2/LConn1 -- Conn1/RConn1
  Conn2/RConn1 -- Rigid Transform1/RConn1
  Rigid Transform2/RConn1 -- Rigid Transform1/LConn1 -- Base/RConn1

== system uncontrolled_case/Double planar manipulator (cable)/Cavo ==
  Brick Solid : sm_lib/Body Elements/Brick Solid  GraphicAmbientColor=[0.15 0.15 0.15 1.0]  BasedOnType=Mass  BrickDimensions=[L W H]  BrickDimensionUnits=m  CenterOfMass=[0 0 0]  CenterOfMassUnits=m  GraphicDiffuseColor=rgb  Density=1000  DensityUnits=kg/m^3  DoExposeReferenceFrame=on  GraphicEmissiveColor=[0.0 0.0 0.0 1.0]  ExportEntireGeometry=off  SerializedFrames=<Frames/>  MarkerShape=Sphere  MarkerSize=10  GraphicType=FromGeometry  InertiaType=CalculateFromGeometry  Mass=m  MassUnits=kg  MomentsOfInertia=[1 1 1]  MomentsOfInertiaUnits=kg*m^2  GraphicOpacity=1.0  ProductsOfInertia=[0 0 0]  ProductsOfInertiaUnits=kg*m^2  GraphicShininess=75  GraphicSpecularColor=[0.5 0.5 0.5 1.0]  GraphicVisPropType=SimpleVisualProperties
  Rigid Transform : sm_lib/Frames and Transforms/Rigid Transform  TranslationMethod=StandardAxis  TranslationStandardOffset=L/2  TranslationLengthUnit=m  TranslationStandardAxis=-X  TranslationCartesianOffset=[0 0 0]  TranslationROffset=0  TranslationROffsetUnits=m  TranslationZOffset=0  TranslationZOffsetUnits=m  TranslationThetaOffset=0  TranslationThetaOffsetUnits=deg  RotationMethod=None  RotationAngleUnits=deg  RotationStandardAxis=+Z  RotationAngle=0.0  RotationArbitraryAxis=[0 0 1]  FollAlignAxisA=+X  BaseAlignAxisA=+Y  FollAlignAxisB=+Y  BaseAlignAxisB=+Z  RotationSequenceAxes=FollowerAxes  RotationSequence=XYX  RotationSequenceAngles=[0 0 0]  RotationSequenceAnglesUnits=deg  RotationMatrix=[1 0 0; 0 1 0; 0 0 1]
  Rigid Transform1 : sm_lib/Frames and Transforms/Rigid Transform  TranslationMethod=StandardAxis  TranslationStandardOffset=L/2  TranslationLengthUnit=m  TranslationStandardAxis=+X  TranslationCartesianOffset=[0 0 0]  TranslationROffset=0  TranslationROffsetUnits=m  TranslationZOffset=0  TranslationZOffsetUnits=m  TranslationThetaOffset=0  TranslationThetaOffsetUnits=deg  RotationMethod=StandardAxis  RotationAngleUnits=deg  RotationStandardAxis=+Z  RotationAngle=90  RotationArbitraryAxis=[0 0 1]  FollAlignAxisA=+X  BaseAlignAxisA=+Y  FollAlignAxisB=+Y  BaseAlignAxisB=+Z  RotationSequenceAxes=FollowerAxes  RotationSequence=XYX  RotationSequenceAngles=[0 0 0]  RotationSequenceAnglesUnits=deg  RotationMatrix=[1 0 0; 0 1 0; 0 0 1]
  Conn1 : PMIOPort  Side=Left
  Conn2 : PMIOPort  Port=2  Side=Right
  connections:
  Rigid Transform1/RConn1 -- Conn2/RConn1
  Rigid Transform/LConn1 -- Brick Solid/RConn1 -- Rigid Transform1/LConn1
  Rigid Transform/RConn1 -- Conn1/RConn1

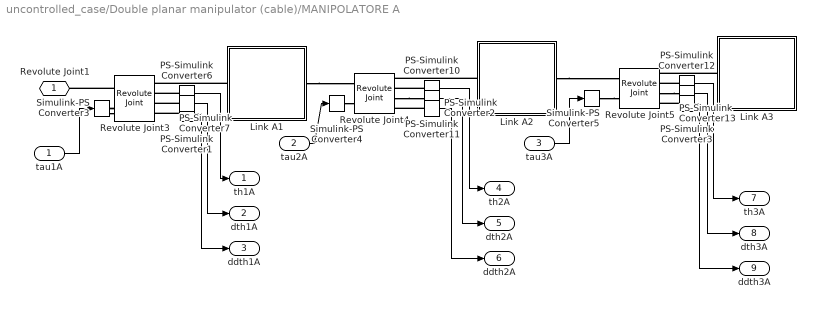
== system uncontrolled_case/Double planar manipulator (cable)/MANIPOLATORE A ==
  tau1A : Inport
  tau2A : Inport  Port=2
  tau3A : Inport  Port=3
  Link A1 : Subsystem  mask{L=a1, W=0.1, H=0.1, m=ml1, rgb=[0.25 0.40 0.70]}
      mask prompts: L "Lenght (m)"; W "Width (m)"; H "Thickness (m)"; m "Mass (kg)"; rgb "Color [R G B]"
  Link A2 : Subsystem  mask{L=a2, W=0.1, H=0.1, m=ml2, rgb=[0.25 0.40 0.70]}
      mask prompts: L "Lenght (m)"; W "Width (m)"; H "Thickness (m)"; m "Mass (kg)"; rgb "Color [R G B]"
  Link A3 : Subsystem  mask{L=a3, W=0.1, H=0.1, m=ml3, rgb=[0.25 0.40 0.70]}
      mask prompts: L "Lenght (m)"; W "Width (m)"; H "Thickness (m)"; m "Mass (kg)"; rgb "Color [R G B]"
  PS-Simulink Converter{1..3,6..7,10..13} (9 alike) : nesl_utility/PS-Simulink Converter  PhysicalDomain=network_engine_domain  SubClassName=ps_output  LeftPortType=input  RightPortType=output  PseudoPeriodic=off  Frequencies=[]  Unit=inherit  AffineConversion=off
  Revolute Joint3 : sm_lib/Joints/Revolute Joint  JointMode=Normal  SenseConstraintForce=off  SenseConstraintForceX=off  SenseConstraintForceY=off  SenseConstraintForceZ=off  SenseConstraintTorque=off  SenseConstraintTorqueX=off  SenseConstraintTorqueY=off  SenseConstraintTorqueZ=off  SenseTotalForce=off  SenseTotalForceX=off  SenseTotalForceY=off  SenseTotalForceZ=off  SenseTotalTorque=off  SenseTotalTorqueX=off  SenseTotalTorqueY=off  SenseTotalTorqueZ=off  CompositeWrenchDir=FollowerOnBase  CompositeWrenchFrame=BaseFrame  EquilibriumPosition=0  EquilibriumPositionUnits=deg  SpringStiffness=0  SpringStiffnessUnits=N*m/deg  DampingCoefficient=fv1  DampingCoefficientUnits=N*m/(rad/s)  TorqueActuationMode=InputTorque  MotionActuationMode=ComputedMotion  SensePosition=on  SenseVelocity=on  SenseAcceleration=on  SenseTorqueForce=off  SenseLowerLimitTorqueForce=off  SenseUpperLimitTorqueForce=off  LowerLimitSpecify=off  LowerLimitBound=-90  LowerLimitBoundUnits=deg  LowerLimitStiffness=1e4  LowerLimitStiffnessUnits=N*m/deg  LowerLimitDamping=10  LowerLimitDampingUnits=N*m/(deg/s)  LowerLimitTransitionRegionWidth=0.1  LowerLimitTransitionRegionWidthUnits=deg  UpperLimitSpecify=off  UpperLimitBound=90  UpperLimitBoundUnits=deg  UpperLimitStiffness=1e4  UpperLimitStiffnessUnits=N*m/deg  UpperLimitDamping=10  UpperLimitDampingUnits=N*m/(deg/s)  UpperLimitTransitionRegionWidth=0.1  UpperLimitTransitionRegionWidthUnits=deg  PositionTargetSpecify=on  PositionTargetPriority=High  PositionTargetValue=th1_0  PositionTargetValueUnits=rad  VelocityTargetSpecify=off  VelocityTargetPriority=High  VelocityTargetValue=0  VelocityTargetValueUnits=deg/s
  Revolute Joint4 : sm_lib/Joints/Revolute Joint  JointMode=Normal  SenseConstraintForce=off  SenseConstraintForceX=off  SenseConstraintForceY=off  SenseConstraintForceZ=off  SenseConstraintTorque=off  SenseConstraintTorqueX=off  SenseConstraintTorqueY=off  SenseConstraintTorqueZ=off  SenseTotalForce=off  SenseTotalForceX=off  SenseTotalForceY=off  SenseTotalForceZ=off  SenseTotalTorque=off  SenseTotalTorqueX=off  SenseTotalTorqueY=off  SenseTotalTorqueZ=off  CompositeWrenchDir=FollowerOnBase  CompositeWrenchFrame=BaseFrame  EquilibriumPosition=0  EquilibriumPositionUnits=deg  SpringStiffness=0  SpringStiffnessUnits=N*m/deg  DampingCoefficient=fv2  DampingCoefficientUnits=N*m/(rad/s)  TorqueActuationMode=InputTorque  MotionActuationMode=ComputedMotion  SensePosition=on  SenseVelocity=on  SenseAcceleration=on  SenseTorqueForce=off  SenseLowerLimitTorqueForce=off  SenseUpperLimitTorqueForce=off  LowerLimitSpecify=off  LowerLimitBound=-90  LowerLimitBoundUnits=deg  LowerLimitStiffness=1e4  LowerLimitStiffnessUnits=N*m/deg  LowerLimitDamping=10  LowerLimitDampingUnits=N*m/(deg/s)  LowerLimitTransitionRegionWidth=0.1  LowerLimitTransitionRegionWidthUnits=deg  UpperLimitSpecify=off  UpperLimitBound=90  UpperLimitBoundUnits=deg  UpperLimitStiffness=1e4  UpperLimitStiffnessUnits=N*m/deg  UpperLimitDamping=10  UpperLimitDampingUnits=N*m/(deg/s)  UpperLimitTransitionRegionWidth=0.1  UpperLimitTransitionRegionWidthUnits=deg  PositionTargetSpecify=on  PositionTargetPriority=High  PositionTargetValue=th2_0  PositionTargetValueUnits=rad  VelocityTargetSpecify=off  VelocityTargetPriority=High  VelocityTargetValue=0  VelocityTargetValueUnits=deg/s
  Revolute Joint5 : sm_lib/Joints/Revolute Joint  JointMode=Normal  SenseConstraintForce=off  SenseConstraintForceX=off  SenseConstraintForceY=off  SenseConstraintForceZ=off  SenseConstraintTorque=off  SenseConstraintTorqueX=off  SenseConstraintTorqueY=off  SenseConstraintTorqueZ=off  SenseTotalForce=off  SenseTotalForceX=off  SenseTotalForceY=off  SenseTotalForceZ=off  SenseTotalTorque=off  SenseTotalTorqueX=off  SenseTotalTorqueY=off  SenseTotalTorqueZ=off  CompositeWrenchDir=FollowerOnBase  CompositeWrenchFrame=BaseFrame  EquilibriumPosition=0  EquilibriumPositionUnits=deg  SpringStiffness=0  SpringStiffnessUnits=N*m/deg  DampingCoefficient=fv3  DampingCoefficientUnits=N*m/(rad/s)  TorqueActuationMode=InputTorque  MotionActuationMode=ComputedMotion  SensePosition=on  SenseVelocity=on  SenseAcceleration=on  SenseTorqueForce=off  SenseLowerLimitTorqueForce=off  SenseUpperLimitTorqueForce=off  LowerLimitSpecify=off  LowerLimitBound=-90  LowerLimitBoundUnits=deg  LowerLimitStiffness=1e4  LowerLimitStiffnessUnits=N*m/deg  LowerLimitDamping=10  LowerLimitDampingUnits=N*m/(deg/s)  LowerLimitTransitionRegionWidth=0.1  LowerLimitTransitionRegionWidthUnits=deg  UpperLimitSpecify=off  UpperLimitBound=90  UpperLimitBoundUnits=deg  UpperLimitStiffness=1e4  UpperLimitStiffnessUnits=N*m/deg  UpperLimitDamping=10  UpperLimitDampingUnits=N*m/(deg/s)  UpperLimitTransitionRegionWidth=0.1  UpperLimitTransitionRegionWidthUnits=deg  PositionTargetSpecify=on  PositionTargetPriority=High  PositionTargetValue=th3_0  PositionTargetValueUnits=rad  VelocityTargetSpecify=off  VelocityTargetPriority=High  VelocityTargetValue=0  VelocityTargetValueUnits=deg/s
  Simulink-PS Converter3 : nesl_utility/Simulink-PS Converter  PhysicalDomain=network_engine_domain  SubClassName=ps_input  LeftPortType=input  RightPortType=output  PseudoPeriodic=off  Frequencies=[]  NoiseDistribution=none  NoiseParameters=[]  Unit=1  AffineConversion=off  FilteringAndDerivatives=provide  SimscapeFilterOrder=1  InputFilterTimeConstant=0.001  UdotUserProvided=0
  Simulink-PS Converter4 : nesl_utility/Simulink-PS Converter  PhysicalDomain=network_engine_domain  SubClassName=ps_input  LeftPortType=input  RightPortType=output  PseudoPeriodic=off  Frequencies=[]  NoiseDistribution=none  NoiseParameters=[]  Unit=1  AffineConversion=off  FilteringAndDerivatives=provide  SimscapeFilterOrder=1  InputFilterTimeConstant=0.001  UdotUserProvided=0
  Simulink-PS Converter5 : nesl_utility/Simulink-PS Converter  PhysicalDomain=network_engine_domain  SubClassName=ps_input  LeftPortType=input  RightPortType=output  PseudoPeriodic=off  Frequencies=[]  NoiseDistribution=none  NoiseParameters=[]  Unit=1  AffineConversion=off  FilteringAndDerivatives=provide  SimscapeFilterOrder=1  InputFilterTimeConstant=0.001  UdotUserProvided=0
  Revolute Joint1 : PMIOPort  Side=Left
  th1A : Outport
  dth1A : Outport  Port=2
  ddth1A : Outport  Port=3
  th2A : Outport  Port=4
  dth2A : Outport  Port=5
  ddth2A : Outport  Port=6
  th3A : Outport  Port=7
  dth3A : Outport  Port=8
  ddth3A : Outport  Port=9
  wires:
  PS-Simulink Converter11/1 -> dth2A/1
  PS-Simulink Converter12/1 -> th3A/1
  PS-Simulink Converter13/1 -> dth3A/1
  tau1A/1 -> Simulink-PS Converter3/1
  tau3A/1 -> Simulink-PS Converter5/1
  tau2A/1 -> Simulink-PS Converter4/1
  PS-Simulink Converter10/1 -> th2A/1
  PS-Simulink Converter6/1 -> th1A/1
  PS-Simulink Converter7/1 -> dth1A/1
  PS-Simulink Converter1/1 -> ddth1A/1
  PS-Simulink Converter2/1 -> ddth2A/1
  PS-Simulink Converter3/1 -> ddth3A/1
  connections:
  PS-Simulink Converter12/LConn1 -- Revolute Joint5/RConn2
  Link A2/RConn1 -- Revolute Joint5/LConn1
  PS-Simulink Converter6/LConn1 -- Revolute Joint3/RConn2
  Revolute Joint4/RConn3 -- PS-Simulink Converter11/LConn1
  Link A1/RConn1 -- Revolute Joint4/LConn1
  Simulink-PS Converter5/RConn1 -- Revolute Joint5/LConn2
  PS-Simulink Converter7/LConn1 -- Revolute Joint3/RConn3
  Simulink-PS Converter4/RConn1 -- Revolute Joint4/LConn2
  Link A1/LConn1 -- Revolute Joint3/RConn1
  Revolute Joint3/LConn1 -- Revolute Joint1/RConn1
  Link A2/LConn1 -- Revolute Joint4/RConn1
  Revolute Joint5/RConn3 -- PS-Simulink Converter13/LConn1
  Link A3/LConn1 -- Revolute Joint5/RConn1
  Simulink-PS Converter3/RConn1 -- Revolute Joint3/LConn2
  PS-Simulink Converter10/LConn1 -- Revolute Joint4/RConn2
  PS-Simulink Converter1/LConn1 -- Revolute Joint3/RConn4
  PS-Simulink Converter2/LConn1 -- Revolute Joint4/RConn4
  PS-Simulink Converter3/LConn1 -- Revolute Joint5/RConn4

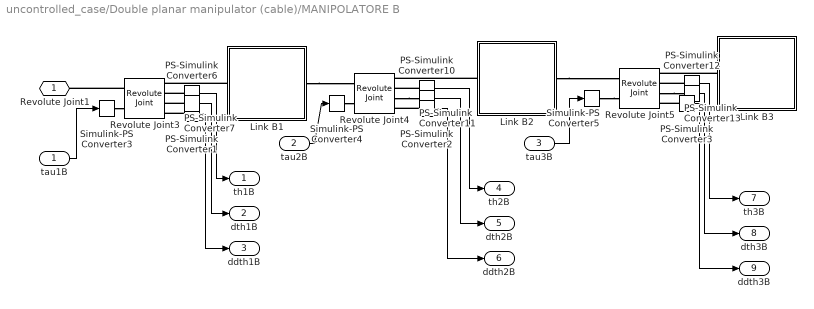
== system uncontrolled_case/Double planar manipulator (cable)/MANIPOLATORE B ==
  tau1B : Inport
  tau2B : Inport  Port=2
  tau3B : Inport  Port=3
  Link B1 : Subsystem  mask{L=a1, W=0.1, H=0.1, m=ml1, rgb=[0.25 0.40 0.70]}
      mask prompts: L "Lenght (m)"; W "Width (m)"; H "Thickness (m)"; m "Mass (kg)"; rgb "Color [R G B]"
  Link B2 : Subsystem  mask{L=a2, W=0.1, H=0.1, m=ml2, rgb=[0.25 0.40 0.70]}
      mask prompts: L "Lenght (m)"; W "Width (m)"; H "Thickness (m)"; m "Mass (kg)"; rgb "Color [R G B]"
  Link B3 : Subsystem  mask{L=a3, W=0.1, H=0.1, m=ml3, rgb=[0.25 0.40 0.70]}
      mask prompts: L "Lenght (m)"; W "Width (m)"; H "Thickness (m)"; m "Mass (kg)"; rgb "Color [R G B]"
  PS-Simulink Converter{1..3,6..7,10..13} (9 alike) : nesl_utility/PS-Simulink Converter  PhysicalDomain=network_engine_domain  SubClassName=ps_output  LeftPortType=input  RightPortType=output  PseudoPeriodic=off  Frequencies=[]  Unit=inherit  AffineConversion=off
  Revolute Joint3 : sm_lib/Joints/Revolute Joint  JointMode=Normal  SenseConstraintForce=off  SenseConstraintForceX=off  SenseConstraintForceY=off  SenseConstraintForceZ=off  SenseConstraintTorque=off  SenseConstraintTorqueX=off  SenseConstraintTorqueY=off  SenseConstraintTorqueZ=off  SenseTotalForce=off  SenseTotalForceX=off  SenseTotalForceY=off  SenseTotalForceZ=off  SenseTotalTorque=off  SenseTotalTorqueX=off  SenseTotalTorqueY=off  SenseTotalTorqueZ=off  CompositeWrenchDir=FollowerOnBase  CompositeWrenchFrame=BaseFrame  EquilibriumPosition=0  EquilibriumPositionUnits=deg  SpringStiffness=0  SpringStiffnessUnits=N*m/deg  DampingCoefficient=fv1  DampingCoefficientUnits=N*m/(rad/s)  TorqueActuationMode=InputTorque  MotionActuationMode=ComputedMotion  SensePosition=on  SenseVelocity=on  SenseAcceleration=on  SenseTorqueForce=off  SenseLowerLimitTorqueForce=off  SenseUpperLimitTorqueForce=off  LowerLimitSpecify=off  LowerLimitBound=-90  LowerLimitBoundUnits=deg  LowerLimitStiffness=1e4  LowerLimitStiffnessUnits=N*m/deg  LowerLimitDamping=10  LowerLimitDampingUnits=N*m/(deg/s)  LowerLimitTransitionRegionWidth=0.1  LowerLimitTransitionRegionWidthUnits=deg  UpperLimitSpecify=off  UpperLimitBound=90  UpperLimitBoundUnits=deg  UpperLimitStiffness=1e4  UpperLimitStiffnessUnits=N*m/deg  UpperLimitDamping=10  UpperLimitDampingUnits=N*m/(deg/s)  UpperLimitTransitionRegionWidth=0.1  UpperLimitTransitionRegionWidthUnits=deg  PositionTargetSpecify=on  PositionTargetPriority=High  PositionTargetValue=th1_0  PositionTargetValueUnits=rad  VelocityTargetSpecify=off  VelocityTargetPriority=High  VelocityTargetValue=0  VelocityTargetValueUnits=deg/s
  Revolute Joint4 : sm_lib/Joints/Revolute Joint  JointMode=Normal  SenseConstraintForce=off  SenseConstraintForceX=off  SenseConstraintForceY=off  SenseConstraintForceZ=off  SenseConstraintTorque=off  SenseConstraintTorqueX=off  SenseConstraintTorqueY=off  SenseConstraintTorqueZ=off  SenseTotalForce=off  SenseTotalForceX=off  SenseTotalForceY=off  SenseTotalForceZ=off  SenseTotalTorque=off  SenseTotalTorqueX=off  SenseTotalTorqueY=off  SenseTotalTorqueZ=off  CompositeWrenchDir=FollowerOnBase  CompositeWrenchFrame=BaseFrame  EquilibriumPosition=0  EquilibriumPositionUnits=deg  SpringStiffness=0  SpringStiffnessUnits=N*m/deg  DampingCoefficient=fv2  DampingCoefficientUnits=N*m/(rad/s)  TorqueActuationMode=InputTorque  MotionActuationMode=ComputedMotion  SensePosition=on  SenseVelocity=on  SenseAcceleration=on  SenseTorqueForce=off  SenseLowerLimitTorqueForce=off  SenseUpperLimitTorqueForce=off  LowerLimitSpecify=off  LowerLimitBound=-90  LowerLimitBoundUnits=deg  LowerLimitStiffness=1e4  LowerLimitStiffnessUnits=N*m/deg  LowerLimitDamping=10  LowerLimitDampingUnits=N*m/(deg/s)  LowerLimitTransitionRegionWidth=0.1  LowerLimitTransitionRegionWidthUnits=deg  UpperLimitSpecify=off  UpperLimitBound=90  UpperLimitBoundUnits=deg  UpperLimitStiffness=1e4  UpperLimitStiffnessUnits=N*m/deg  UpperLimitDamping=10  UpperLimitDampingUnits=N*m/(deg/s)  UpperLimitTransitionRegionWidth=0.1  UpperLimitTransitionRegionWidthUnits=deg  PositionTargetSpecify=on  PositionTargetPriority=High  PositionTargetValue=th2_0  PositionTargetValueUnits=rad  VelocityTargetSpecify=off  VelocityTargetPriority=High  VelocityTargetValue=0  VelocityTargetValueUnits=deg/s
  Revolute Joint5 : sm_lib/Joints/Revolute Joint  JointMode=Normal  SenseConstraintForce=off  SenseConstraintForceX=off  SenseConstraintForceY=off  SenseConstraintForceZ=off  SenseConstraintTorque=off  SenseConstraintTorqueX=off  SenseConstraintTorqueY=off  SenseConstraintTorqueZ=off  SenseTotalForce=off  SenseTotalForceX=off  SenseTotalForceY=off  SenseTotalForceZ=off  SenseTotalTorque=off  SenseTotalTorqueX=off  SenseTotalTorqueY=off  SenseTotalTorqueZ=off  CompositeWrenchDir=FollowerOnBase  CompositeWrenchFrame=BaseFrame  EquilibriumPosition=0  EquilibriumPositionUnits=deg  SpringStiffness=0  SpringStiffnessUnits=N*m/deg  DampingCoefficient=fv3  DampingCoefficientUnits=N*m/(rad/s)  TorqueActuationMode=InputTorque  MotionActuationMode=ComputedMotion  SensePosition=on  SenseVelocity=on  SenseAcceleration=on  SenseTorqueForce=off  SenseLowerLimitTorqueForce=off  SenseUpperLimitTorqueForce=off  LowerLimitSpecify=off  LowerLimitBound=-90  LowerLimitBoundUnits=deg  LowerLimitStiffness=1e4  LowerLimitStiffnessUnits=N*m/deg  LowerLimitDamping=10  LowerLimitDampingUnits=N*m/(deg/s)  LowerLimitTransitionRegionWidth=0.1  LowerLimitTransitionRegionWidthUnits=deg  UpperLimitSpecify=off  UpperLimitBound=90  UpperLimitBoundUnits=deg  UpperLimitStiffness=1e4  UpperLimitStiffnessUnits=N*m/deg  UpperLimitDamping=10  UpperLimitDampingUnits=N*m/(deg/s)  UpperLimitTransitionRegionWidth=0.1  UpperLimitTransitionRegionWidthUnits=deg  PositionTargetSpecify=on  PositionTargetPriority=High  PositionTargetValue=th3_0  PositionTargetValueUnits=rad  VelocityTargetSpecify=off  VelocityTargetPriority=High  VelocityTargetValue=0  VelocityTargetValueUnits=deg/s
  Simulink-PS Converter3 : nesl_utility/Simulink-PS Converter  PhysicalDomain=network_engine_domain  SubClassName=ps_input  LeftPortType=input  RightPortType=output  PseudoPeriodic=off  Frequencies=[]  NoiseDistribution=none  NoiseParameters=[]  Unit=1  AffineConversion=off  FilteringAndDerivatives=provide  SimscapeFilterOrder=1  InputFilterTimeConstant=0.001  UdotUserProvided=0
  Simulink-PS Converter4 : nesl_utility/Simulink-PS Converter  PhysicalDomain=network_engine_domain  SubClassName=ps_input  LeftPortType=input  RightPortType=output  PseudoPeriodic=off  Frequencies=[]  NoiseDistribution=none  NoiseParameters=[]  Unit=1  AffineConversion=off  FilteringAndDerivatives=provide  SimscapeFilterOrder=1  InputFilterTimeConstant=0.001  UdotUserProvided=0
  Simulink-PS Converter5 : nesl_utility/Simulink-PS Converter  PhysicalDomain=network_engine_domain  SubClassName=ps_input  LeftPortType=input  RightPortType=output  PseudoPeriodic=off  Frequencies=[]  NoiseDistribution=none  NoiseParameters=[]  Unit=1  AffineConversion=off  FilteringAndDerivatives=provide  SimscapeFilterOrder=1  InputFilterTimeConstant=0.001  UdotUserProvided=0
  Revolute Joint1 : PMIOPort  Side=Left
  th1B : Outport
  dth1B : Outport  Port=2
  ddth1B : Outport  Port=3
  th2B : Outport  Port=4
  dth2B : Outport  Port=5
  ddth2B : Outport  Port=6
  th3B : Outport  Port=7
  dth3B : Outport  Port=8
  ddth3B : Outport  Port=9
  wires:
  PS-Simulink Converter11/1 -> dth2B/1
  PS-Simulink Converter12/1 -> th3B/1
  PS-Simulink Converter13/1 -> dth3B/1
  tau1B/1 -> Simulink-PS Converter3/1
  tau3B/1 -> Simulink-PS Converter5/1
  tau2B/1 -> Simulink-PS Converter4/1
  PS-Simulink Converter10/1 -> th2B/1
  PS-Simulink Converter6/1 -> th1B/1
  PS-Simulink Converter7/1 -> dth1B/1
  PS-Simulink Converter1/1 -> ddth1B/1
  PS-Simulink Converter2/1 -> ddth2B/1
  PS-Simulink Converter3/1 -> ddth3B/1
  connections:
  PS-Simulink Converter12/LConn1 -- Revolute Joint5/RConn2
  Link B2/RConn1 -- Revolute Joint5/LConn1
  PS-Simulink Converter6/LConn1 -- Revolute Joint3/RConn2
  Revolute Joint4/RConn3 -- PS-Simulink Converter11/LConn1
  Link B1/RConn1 -- Revolute Joint4/LConn1
  Simulink-PS Converter5/RConn1 -- Revolute Joint5/LConn2
  PS-Simulink Converter7/LConn1 -- Revolute Joint3/RConn3
  Simulink-PS Converter4/RConn1 -- Revolute Joint4/LConn2
  Link B1/LConn1 -- Revolute Joint3/RConn1
  Revolute Joint3/LConn1 -- Revolute Joint1/RConn1
  Link B2/LConn1 -- Revolute Joint4/RConn1
  Revolute Joint5/RConn3 -- PS-Simulink Converter13/LConn1
  Link B3/LConn1 -- Revolute Joint5/RConn1
  Simulink-PS Converter3/RConn1 -- Revolute Joint3/LConn2
  PS-Simulink Converter10/LConn1 -- Revolute Joint4/RConn2
  PS-Simulink Converter1/LConn1 -- Revolute Joint3/RConn4
  PS-Simulink Converter2/LConn1 -- Revolute Joint4/RConn4
  PS-Simulink Converter3/LConn1 -- Revolute Joint5/RConn4
